simulink model "fcn"  (R2020b)
settings: Solver=VariableStepAuto  StartTime=0.0  StopTime=10.0  RelTol=1e-3
StartFcn:
  | learning.simulink.clearGlows(gcs);learning.simulink.resetGraderBadge(gcs);learning.simulink.closeNotificationBar(gcs);learning.simulink.Application.getInstance().clearStateflowBreakpoints()
StopFcn:
  | save_system(gcs);learning.simulink.refreshSignalWindows
model workspace (MAT data in the model file):
  courseObject.course = 'simulink'
  courseObject.chapter = 7
  courseObject.lesson = 2
  courseObject.section = 2
  courseObject.task = 1
  t_ans = [0; 0.1; 0.2; 0.3; 0.4; 0.5; 0.6; 0.7; 0.8; 0.9; 1; 1.1; 1.2; 1.3; 1.4; 1.5; 1.6; 1.7; 1.8; 1.9; 2; 2.1; 2.2; 2.3; 2.4; 2.5; 2.6; 2.7; 2.8; 2.9; 3; 3.1; 3.2; 3.3; 3.4; 3.5; 3.6; 3.7; 3.8; 3.9; 4; 4.1; 4.2; 4.3; 4.4; 4.5; 4.6; 4.7; 4.8; 4.9; 5; 5.1; 5.2; 5.3; 5.4; 5.5; 5.6; 5.7; 5.8; 5.9; 6; 6.1; 6.2; 6.3; 6.4; 6.5; 6.6; 6.7; 6.8; 6.9; 7; 7.1; 7.2; 7.3; 7.4; 7.5; 7.6; 7.7; 7.8; 7.9; 8; 8.1; 8.2; 8.3; 8.4; 8.5; 8.6; 8.7; 8.8; 8.9; 9; 9.1; 9.2; 9.3; 9.4; 9.5; 9.6; 9.7; 9.8; 9.9; 10]
  y_ans = [0; 34674.6328174; 97890.8777522; 179275.304306; 274804.958264; 381890.002573; 498550.428358; 623125.29792; 754141.649649; 890247.144713; 1030172.77485; 1172711.42001; 1316705.45914; 1461039.86821; 1604638.79406; 1746464.40107; 1885517.23383; 2020837.59912; 2151507.62815; 2276653.77947; 2395449.60779; 2507118.66764; 2610937.45095; 2706238.27907; 2792412.08566; 2868911.03872; 2935250.95932; 2991013.50225; 3035848.06955; 3069473.43386; 3091679.05256; 3102326.05837; 3101347.91565; 3088750.73577; 3064613.2481; 3029086.42703; 2982392.77886; 2924825.29591; 2856746.08932; 2778584.71548; 2690836.21576; 2594058.89367; 2488871.85939; 2375952.37741; 2256033.06142; 2129898.96982; 1998384.66776; 1862371.33845; 1722784.04883; 1580589.30711; 1436793.09602; 1292439.63508; 1148611.23256; 1006429.75899; 867060.557323; 731720.096988; 601689.576482; 478338.427163; 363165.357474; 257873.205636; 164517.162306; 85843.6511429; 26312.7007691; 2392.26375228; 43768.2419269; 110443.43814; 194430.58876; 292062.141297; 400884.685804; 518985.784411; 644742.874069; 776706.903351; 913541.601181; 1053989.55776; 1196852.65986; 1340980.8176; 1485265.75919; 1628638.0557; 1770066.26676; 1908557.50407; 2043158.94829; 2172959.99995; 2297094.8379; 2414745.21905; 2525143.3941; 2627575.04252; 2721382.1503; 2805965.76913; 2880788.60702; 2945377.40922; 2999325.09581; 3042292.62796; 3074010.5805; 3094280.40249; 3102975.35231; 3100041.097; 3085495.96984; 3059430.88341; 3022008.899; 2973464.45696; 2914102.27594]
CloseFcn:
  | learning.simulink.cleanupOnlineTraining
settings Model: Creator=vvikk  LastModifiedBy=vvikk
settings DataIOCC: SaveTime=off

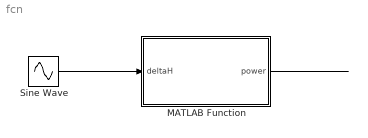
== system fcn ==
  MATLAB Function : MATLAB Function  TreatAsAtomicUnit=on
  Sine Wave : Sin  Amplitude=.75  Frequency=0.5  SampleTime=0
  wires:
  Sine Wave/1 -> MATLAB Function/1(deltaH)
  MATLAB Function/1(power) -> ?

== matlab function fcn/MATLAB Function ==
  data: deltaH input; power output
function power = fcn(deltaH)

Cp = 0.35; % Power coefficient
rho = 1000; % Density of water, kg/m^3
A = pi*10^2; % Area of turbine blade
g = 9.81; % Acceleration of gravity, m/s^2


% Replace the equation below with the correct equation for power
power = 0.5*Cp*rho*A*(2*g*abs(deltaH))^(3/2);
